simulink model "PC_MSFS_STATION"  (R2021b)
settings: Solver=FixedStepAuto  StartTime=0.0  StopTime=2000  FixedStep=0.03  RelTol=1e-3
undefined symbols (not defined in the file): DiscIntNeverNeededParam, f, MODEL, MODEL_INI
libraries: SimConnectToolbox x11, instrumentlib x7, simulink x5
(part 1 of 2)
settings Model: Creator=Andreas  LastModifiedBy=ccortes9
settings SolverCC: AlgebraicLoopSolver=TrustRegion
settings DebuggingCC: InheritedTsInSrcMsg=none  SFMachineParentedDataDiag=warning

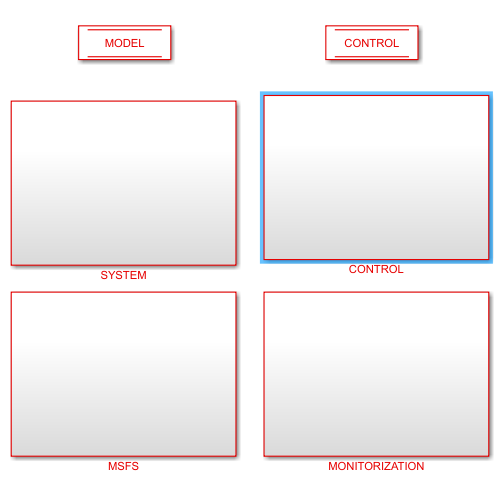
[thumbnail: Simulink's stored preview of the top-level diagram]
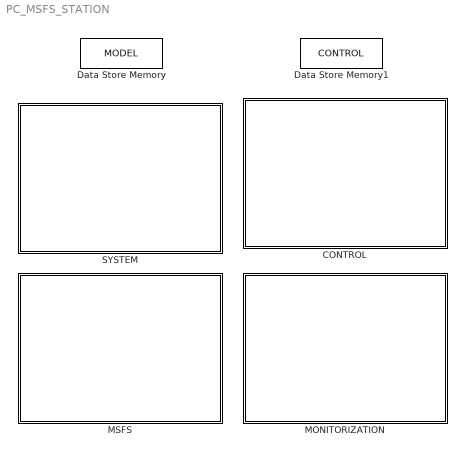
== system PC_MSFS_STATION ==
  CONTROL : Subsystem
  Data Store Memory : DataStoreMemory  DataStoreName=MODEL  ReadBeforeWriteMsg=warning  WriteAfterWriteMsg=warning  WriteAfterReadMsg=warning  InitialValue=MODEL_INI  ShowAdditionalParam=off  OutDataTypeStr=Bus: MODEL_Bus
  Data Store Memory1 : DataStoreMemory  DataStoreName=CONTROL  ReadBeforeWriteMsg=warning  WriteAfterWriteMsg=warning  WriteAfterReadMsg=warning  InitialValue=CONTROL_INI  ShowAdditionalParam=off  OutDataTypeStr=Bus: CONTROL_Bus
  MONITORIZATION : Subsystem
  MSFS : Subsystem
  SYSTEM : Subsystem

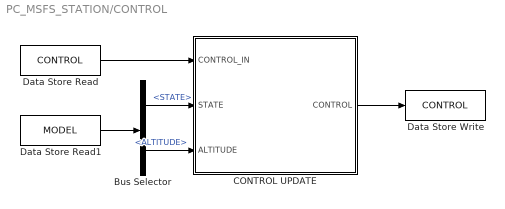
== system PC_MSFS_STATION/CONTROL ==
  Bus Selector : BusSelector  OutputSignals=STATE,INPUT.ALTITUDE
  CONTROL UPDATE : MATLAB Function  TreatAsAtomicUnit=on
  Data Store Read : DataStoreRead  DataStoreName=CONTROL  SampleTime=MODEL_INI.PARAM.SIM_SAMPLING_TIME  IndexOptions=Index vector (dialog)  Indices=1  OutputSizes=1
  Data Store Read1 : DataStoreRead  DataStoreName=MODEL  SampleTime=MODEL_INI.PARAM.SIM_SAMPLING_TIME  IndexOptions=Index vector (dialog)  Indices=1  OutputSizes=1
  Data Store Write : DataStoreWrite  DataStoreName=CONTROL  IndexOptions=Index vector (dialog)  Indices=1  OutputSizes=1
  wires:
  Data Store Read/1 -> CONTROL UPDATE/1(CONTROL_IN)
  CONTROL UPDATE/1(CONTROL) -> Data Store Write/1
  Bus Selector/1 -> CONTROL UPDATE/2(STATE)  "<STATE>"
  Data Store Read1/1 -> Bus Selector/1
  Bus Selector/2 -> CONTROL UPDATE/3(ALTITUDE)  "<ALTITUDE>"

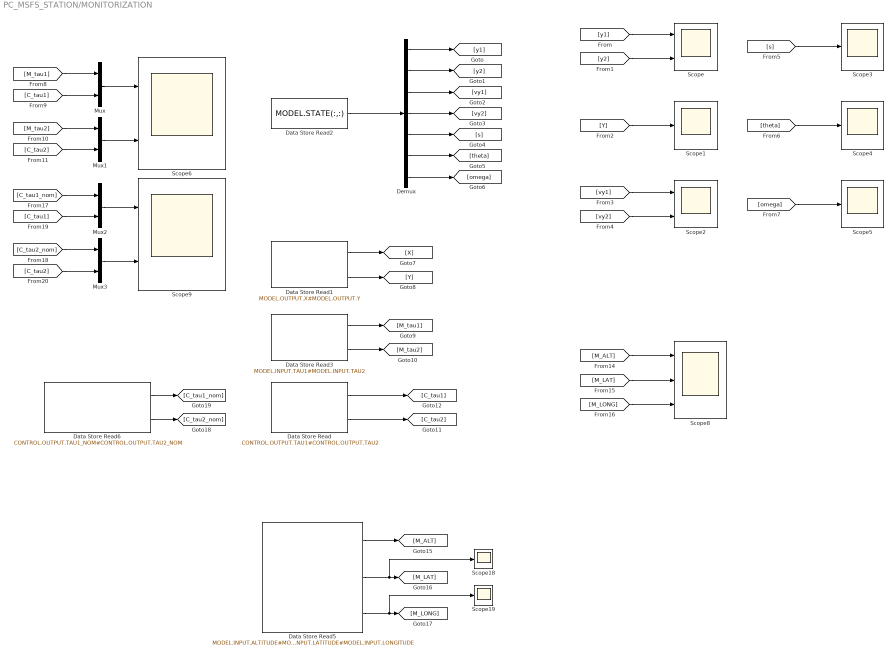
== system PC_MSFS_STATION/MONITORIZATION ==
  Data Store Read : DataStoreRead  DataStoreName=CONTROL  DataStoreElements=CONTROL.OUTPUT.TAU1#CONTROL.OUTPUT.TAU2  IndexOptions=Index vector (dialog)  Indices=1  OutputSizes=1
  Data Store Read1 : DataStoreRead  DataStoreName=MODEL  SampleTime=MODEL_INI.PARAM.SIM_SAMPLING_TIME  DataStoreElements=MODEL.OUTPUT.X#MODEL.OUTPUT.Y  IndexOptions=Index vector (dialog)  Indices=1  OutputSizes=1
  Data Store Read2 : DataStoreRead  DataStoreName=MODEL  SampleTime=MODEL_INI.PARAM.SIM_SAMPLING_TIME  DataStoreElements=MODEL.STATE(:,:)  IndexOptions=Index vector (dialog)  Indices=1  OutputSizes=1
  Data Store Read3 : DataStoreRead  DataStoreName=MODEL  SampleTime=MODEL_INI.PARAM.SIM_SAMPLING_TIME  DataStoreElements=MODEL.INPUT.TAU1#MODEL.INPUT.TAU2  IndexOptions=Index vector (dialog)  Indices=1  OutputSizes=1
  Data Store Read5 : DataStoreRead  DataStoreName=MODEL  SampleTime=MODEL_INI.PARAM.SIM_SAMPLING_TIME  DataStoreElements=MODEL.INPUT.ALTITUDE#MODEL.INPUT.LATITUDE#MODEL.INPUT.LONGITUDE  IndexOptions=Index vector (dialog)  Indices=1  OutputSizes=1
  Data Store Read6 : DataStoreRead  DataStoreName=CONTROL  DataStoreElements=CONTROL.OUTPUT.TAU1_NOM#CONTROL.OUTPUT.TAU2_NOM  IndexOptions=Index vector (dialog)  Indices=1  OutputSizes=1
  Demux : Demux  Outputs=7
  Mux{,1..3} (4 alike) : Mux  Inputs=2
  Scope{,2,6,9} (4 alike) : Scope  NumInputPorts=2
  Scope{1,3..5,18..19} (6 alike) : Scope
  Scope8 : Scope  NumInputPorts=3
  wires:
  Data Store Read2/1 -> Demux/1
  Demux/1 -> [y1]
  Demux/2 -> [y2]
  Demux/3 -> [vy1]
  Demux/4 -> [vy2]
  Demux/5 -> [s]
  Demux/6 -> [theta]
  Demux/7 -> [omega]
  [y1] -> Scope/1
  [y2] -> Scope/2
  Data Store Read1/1 -> [X]
  Data Store Read1/2 -> [Y]
  [Y] -> Scope1/1
  [vy2] -> Scope2/2
  [vy1] -> Scope2/1
  [s] -> Scope3/1
  [theta] -> Scope4/1
  [omega] -> Scope5/1
  Data Store Read3/1 -> [M_tau1]
  Data Store Read3/2 -> [M_tau2]
  Data Store Read/1 -> [C_tau1]
  Data Store Read/2 -> [C_tau2]
  Mux/1 -> Scope6/1
  Mux1/1 -> Scope6/2
  [M_tau1] -> Mux/1
  [M_tau2] -> Mux1/1
  [C_tau2] -> Mux1/2
  [C_tau1] -> Mux/2
  Data Store Read5/2 -> Scope18/1, [M_LAT]
  Data Store Read5/1 -> [M_ALT]
  Data Store Read5/3 -> Scope19/1, [M_LONG]
  [M_LAT] -> Scope8/2
  [M_ALT] -> Scope8/1
  [M_LONG] -> Scope8/3
  Data Store Read6/2 -> [C_tau2_nom]
  Data Store Read6/1 -> [C_tau1_nom]
  [C_tau1] -> Mux2/2
  [C_tau2] -> Mux3/2
  [C_tau2_nom] -> Mux3/1
  [C_tau1_nom] -> Mux2/1
  Mux3/1 -> Scope9/2
  Mux2/1 -> Scope9/1

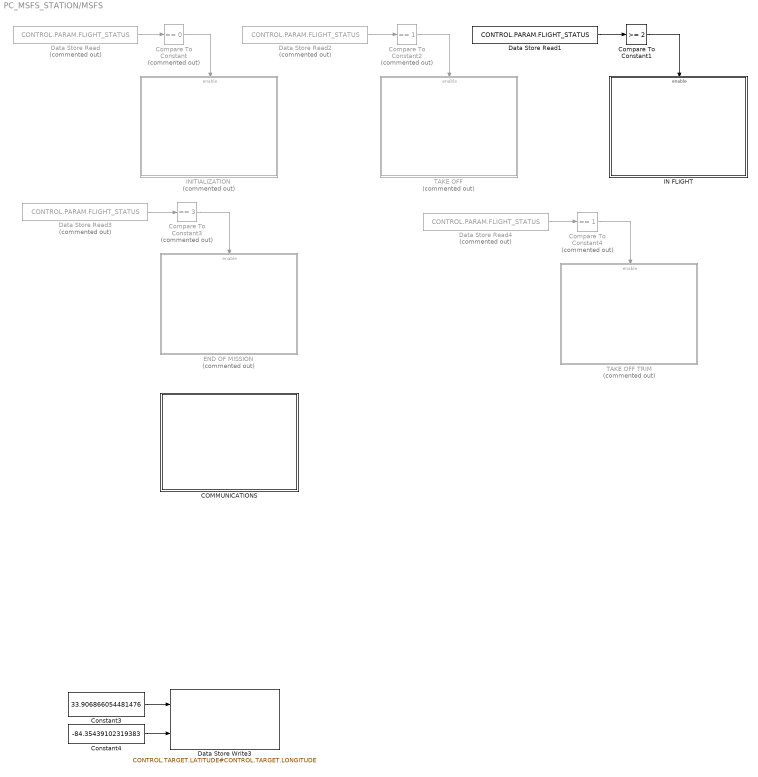
== system PC_MSFS_STATION/MSFS ==
  COMMUNICATIONS : Subsystem
  Compare To Constant : simulink/Logic and Bit Operations/Compare To Constant  Commented=on  relop===  const=0  OutDataTypeStr=boolean
  Compare To Constant1 : simulink/Logic and Bit Operations/Compare To Constant  relop=>=  const=2  OutDataTypeStr=boolean
  Compare To Constant2 : simulink/Logic and Bit Operations/Compare To Constant  Commented=on  relop===  const=1  OutDataTypeStr=boolean
  Compare To Constant3 : simulink/Logic and Bit Operations/Compare To Constant  Commented=on  relop===  const=3  OutDataTypeStr=boolean
  Compare To Constant4 : simulink/Logic and Bit Operations/Compare To Constant  Commented=on  relop===  const=1  OutDataTypeStr=boolean
  Constant3 : Constant  Value=33.906866054481476  SampleTime=-1
  Constant4 : Constant  Value=-84.35439102319383  SampleTime=-1
  Data Store Read{,2..4} (4 alike) : DataStoreRead  Commented=on  DataStoreName=CONTROL  DataStoreElements=CONTROL.PARAM.FLIGHT_STATUS  IndexOptions=Index vector (dialog)  Indices=1  OutputSizes=1
  Data Store Read1 : DataStoreRead  DataStoreName=CONTROL  DataStoreElements=CONTROL.PARAM.FLIGHT_STATUS  IndexOptions=Index vector (dialog)  Indices=1  OutputSizes=1
  Data Store Write3 : DataStoreWrite  DataStoreName=CONTROL  DataStoreElements=CONTROL.TARGET.LATITUDE#CONTROL.TARGET.LONGITUDE  IndexOptions=Index vector (dialog)  Indices=1  OutputSizes=1
  END OF MISSION : Subsystem  Commented=on
  IN FLIGHT : Subsystem
  INITIALIZATION : Subsystem  Commented=on
  TAKE OFF : Subsystem  Commented=on
  TAKE OFF TRIM : Subsystem  Commented=on
  wires:
  Data Store Read/1 -> Compare To Constant/1
  Compare To Constant/1 -> INITIALIZATION/Enable
  Data Store Read1/1 -> Compare To Constant1/1
  Data Store Read2/1 -> Compare To Constant2/1
  Compare To Constant2/1 -> TAKE OFF/Enable
  Compare To Constant3/1 -> END OF MISSION/Enable
  Data Store Read3/1 -> Compare To Constant3/1
  Data Store Read4/1 -> Compare To Constant4/1
  Compare To Constant4/1 -> TAKE OFF TRIM/Enable
  Constant3/1 -> Data Store Write3/1
  Constant4/1 -> Data Store Write3/2
  Compare To Constant1/1 -> IN FLIGHT/Enable

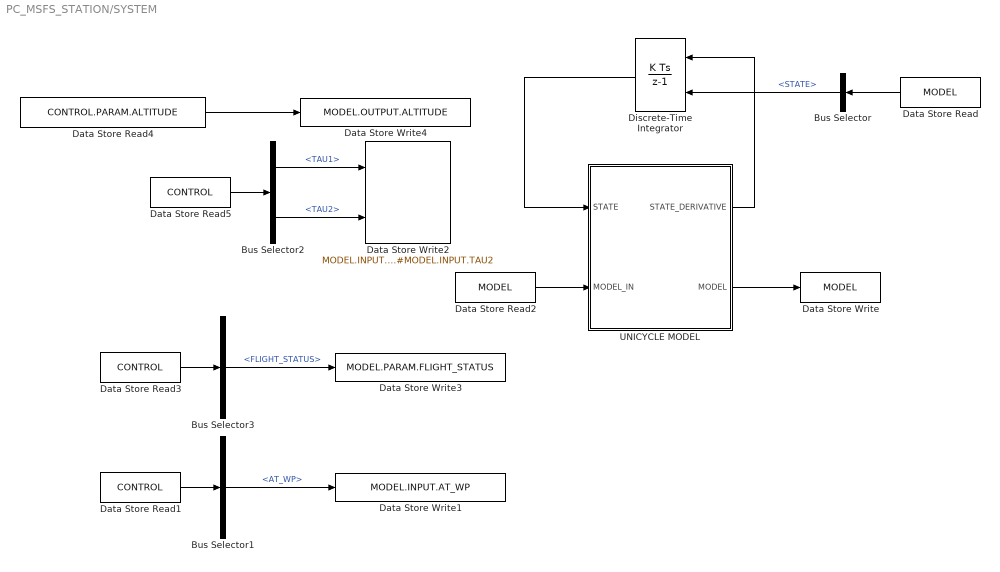
== system PC_MSFS_STATION/SYSTEM ==
  Bus Selector : BusSelector  OutputSignals=STATE
  Bus Selector1 : BusSelector  OutputSignals=OUTPUT.AT_WP
  Bus Selector2 : BusSelector  OutputSignals=OUTPUT.TAU1,OUTPUT.TAU2
  Bus Selector3 : BusSelector  OutputSignals=PARAM.FLIGHT_STATUS
  Data Store Read : DataStoreRead  DataStoreName=MODEL  SampleTime=MODEL_INI.PARAM.SIM_SAMPLING_TIME  IndexOptions=Index vector (dialog)  Indices=1  OutputSizes=1
  Data Store Read1 : DataStoreRead  DataStoreName=CONTROL  IndexOptions=Index vector (dialog)  Indices=1  OutputSizes=1
  Data Store Read2 : DataStoreRead  DataStoreName=MODEL  SampleTime=MODEL_INI.PARAM.SIM_SAMPLING_TIME  IndexOptions=Index vector (dialog)  Indices=1  OutputSizes=1
  Data Store Read3 : DataStoreRead  DataStoreName=CONTROL  IndexOptions=Index vector (dialog)  Indices=1  OutputSizes=1
  Data Store Read4 : DataStoreRead  DataStoreName=CONTROL  DataStoreElements=CONTROL.PARAM.ALTITUDE  IndexOptions=Index vector (dialog)  Indices=1  OutputSizes=1
  Data Store Read5 : DataStoreRead  DataStoreName=CONTROL  IndexOptions=Index vector (dialog)  Indices=1  OutputSizes=1
  Data Store Write : DataStoreWrite  DataStoreName=MODEL  IndexOptions=Index vector (dialog)  Indices=1  OutputSizes=1
  Data Store Write1 : DataStoreWrite  DataStoreName=MODEL  DataStoreElements=MODEL.INPUT.AT_WP  IndexOptions=Index vector (dialog)  Indices=1  OutputSizes=1
  Data Store Write2 : DataStoreWrite  DataStoreName=MODEL  DataStoreElements=MODEL.INPUT.TAU1#MODEL.INPUT.TAU2  IndexOptions=Index vector (dialog)  Indices=1  OutputSizes=1
  Data Store Write3 : DataStoreWrite  DataStoreName=MODEL  DataStoreElements=MODEL.PARAM.FLIGHT_STATUS  IndexOptions=Index vector (dialog)  Indices=1  OutputSizes=1
  Data Store Write4 : DataStoreWrite  DataStoreName=MODEL  DataStoreElements=MODEL.OUTPUT.ALTITUDE  IndexOptions=Index vector (dialog)  Indices=1  OutputSizes=1
  Discrete-Time Integrator : DiscreteIntegrator  InitialConditionSource=external  SampleTime=-1  ICPrevOutput=DiscIntNeverNeededParam  ICPrevScaledInput=DiscIntNeverNeededParam
  UNICYCLE MODEL : MATLAB Function  TreatAsAtomicUnit=on
  wires:
  Discrete-Time Integrator/1 -> UNICYCLE MODEL/1(STATE)
  UNICYCLE MODEL/1(STATE_DERIVATIVE) -> Discrete-Time Integrator/1
  Bus Selector/1 -> Discrete-Time Integrator/2  "<STATE>"
  Data Store Read/1 -> Bus Selector/1
  Data Store Read2/1 -> UNICYCLE MODEL/2(MODEL_IN)
  UNICYCLE MODEL/2(MODEL) -> Data Store Write/1
  Bus Selector2/2 -> Data Store Write2/2  "<TAU2>"
  Bus Selector2/1 -> Data Store Write2/1  "<TAU1>"
  Data Store Read5/1 -> Bus Selector2/1
  Data Store Read3/1 -> Bus Selector3/1
  Bus Selector3/1 -> Data Store Write3/1  "<FLIGHT_STATUS>"
  Data Store Read4/1 -> Data Store Write4/1
  Bus Selector1/1 -> Data Store Write1/1  "<AT_WP>"
  Data Store Read1/1 -> Bus Selector1/1

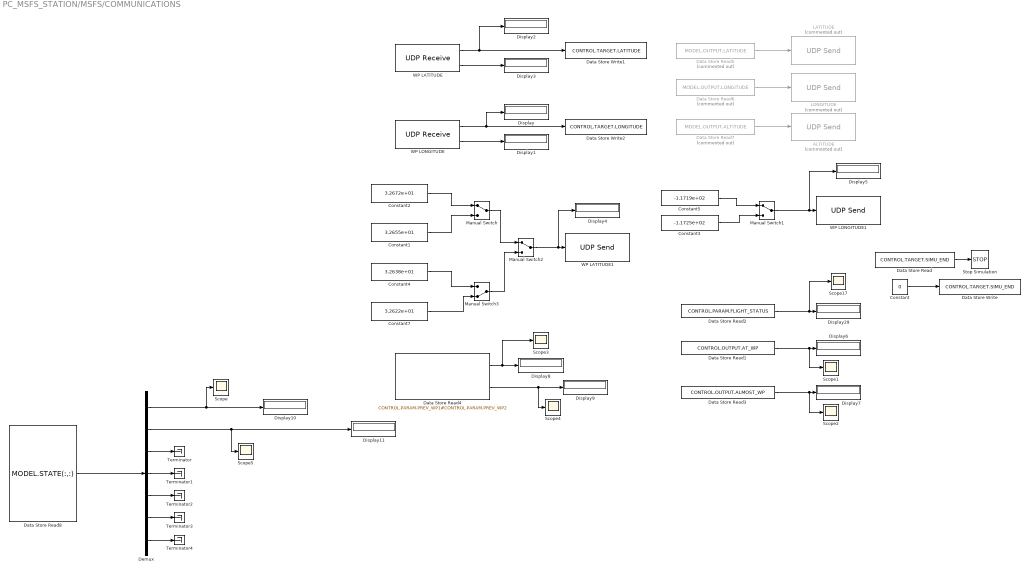
== system PC_MSFS_STATION/MSFS/COMMUNICATIONS ==
  ALTITUDE : instrumentlib/UDP Send  Commented=on  Host=127.0.0.1  Port=8082  LocalPort=8085  EnablePortSharing=off  ByteOrder=BigEndian  OutputDatagramPacketSize=512  EnableBlockingMode=on  LocalAddress=127.0.0.1
  Constant : Constant  Value=0  SampleTime=-1
  Constant1 : Constant  Value=3.2655e+01  SampleTime=0.03
  Constant2 : Constant  Value=3.2672e+01  SampleTime=0.03
  Constant3 : Constant  Value=-1.1725e+02  SampleTime=0.03
  Constant4 : Constant  Value=3.2638e+01  SampleTime=0.03
  Constant5 : Constant  Value=-1.1719e+02  SampleTime=0.03
  Constant7 : Constant  Value=3.2622e+01  SampleTime=0.03
  Data Store Read : DataStoreRead  DataStoreName=CONTROL  DataStoreElements=CONTROL.TARGET.SIMU_END  IndexOptions=Index vector (dialog)  Indices=1  OutputSizes=1
  Data Store Read1 : DataStoreRead  DataStoreName=CONTROL  DataStoreElements=CONTROL.OUTPUT.AT_WP  IndexOptions=Index vector (dialog)  Indices=1  OutputSizes=1
  Data Store Read2 : DataStoreRead  DataStoreName=CONTROL  DataStoreElements=CONTROL.PARAM.FLIGHT_STATUS  IndexOptions=Index vector (dialog)  Indices=1  OutputSizes=1
  Data Store Read3 : DataStoreRead  DataStoreName=CONTROL  DataStoreElements=CONTROL.OUTPUT.ALMOST_WP  IndexOptions=Index vector (dialog)  Indices=1  OutputSizes=1
  Data Store Read4 : DataStoreRead  DataStoreName=CONTROL  DataStoreElements=CONTROL.PARAM.PREV_WP1#CONTROL.PARAM.PREV_WP2  IndexOptions=Index vector (dialog)  Indices=1  OutputSizes=1
  Data Store Read5 : DataStoreRead  Commented=on  DataStoreName=MODEL  DataStoreElements=MODEL.OUTPUT.LATITUDE  IndexOptions=Index vector (dialog)  Indices=1  OutputSizes=1
  Data Store Read6 : DataStoreRead  Commented=on  DataStoreName=MODEL  DataStoreElements=MODEL.OUTPUT.LONGITUDE  IndexOptions=Index vector (dialog)  Indices=1  OutputSizes=1
  Data Store Read7 : DataStoreRead  Commented=on  DataStoreName=MODEL  DataStoreElements=MODEL.OUTPUT.ALTITUDE  IndexOptions=Index vector (dialog)  Indices=1  OutputSizes=1
  Data Store Read8 : DataStoreRead  DataStoreName=MODEL  SampleTime=MODEL_INI.PARAM.SIM_SAMPLING_TIME  DataStoreElements=MODEL.STATE(:,:)  IndexOptions=Index vector (dialog)  Indices=1  OutputSizes=1
  Data Store Write : DataStoreWrite  DataStoreName=CONTROL  DataStoreElements=CONTROL.TARGET.SIMU_END  IndexOptions=Index vector (dialog)  Indices=1  OutputSizes=1
  Data Store Write1 : DataStoreWrite  DataStoreName=CONTROL  DataStoreElements=CONTROL.TARGET.LATITUDE  IndexOptions=Index vector (dialog)  Indices=1  OutputSizes=1
  Data Store Write2 : DataStoreWrite  DataStoreName=CONTROL  DataStoreElements=CONTROL.TARGET.LONGITUDE  IndexOptions=Index vector (dialog)  Indices=1  OutputSizes=1
  Demux : Demux  Outputs=7
  Display{,1..11,29} (13 alike) : Display
  LATITUDE : instrumentlib/UDP Send  Commented=on  Host=127.0.0.1  Port=8086  LocalPort=8081  EnablePortSharing=off  ByteOrder=BigEndian  OutputDatagramPacketSize=512  EnableBlockingMode=on  LocalAddress=127.0.0.1
  LONGITUDE : instrumentlib/UDP Send  Commented=on  Host=127.0.0.1  Port=8084  LocalPort=8083  EnablePortSharing=off  ByteOrder=BigEndian  OutputDatagramPacketSize=512  EnableBlockingMode=on  LocalAddress=127.0.0.1
  Manual Switch : ManualSwitch
  Manual Switch1 : ManualSwitch
  Manual Switch2 : ManualSwitch
  Manual Switch3 : ManualSwitch  CurrentSetting=0
  Scope{,1..5,17} (7 alike) : Scope
  Stop Simulation : Stop
  Terminator{,1..4} (5 alike) : Terminator
  WP LATITUDE : instrumentlib/UDP Receive  Host=127.0.0.1  Port=8087  LocalPort=8080  EnablePortSharing=off  GetLatestData=off  DataSize=[1 1]  DataType=double  ASCIIFormatting=%f,  Terminator=LF  ByteOrder=BigEndian  EnableBlockingMode=off  Timeout=10  SampleTime=-1  LocalAddress=127.0.0.1
  WP LATITUDE1 : instrumentlib/UDP Send  Host=127.0.0.1  Port=8080  LocalPort=8087  EnablePortSharing=off  ByteOrder=BigEndian  OutputDatagramPacketSize=512  EnableBlockingMode=on  LocalAddress=127.0.0.1
  WP LONGITUDE : instrumentlib/UDP Receive  Host=127.0.0.1  Port=8089  LocalPort=8088  EnablePortSharing=off  GetLatestData=off  DataSize=[1 1]  DataType=double  ASCIIFormatting=%f,  Terminator=LF  ByteOrder=BigEndian  EnableBlockingMode=off  Timeout=10  SampleTime=-1  LocalAddress=127.0.0.1
  WP LONGITUDE1 : instrumentlib/UDP Send  Host=127.0.0.1  Port=8088  LocalPort=8089  EnablePortSharing=off  ByteOrder=BigEndian  OutputDatagramPacketSize=512  EnableBlockingMode=on  LocalAddress=127.0.0.1
  wires:
  WP LONGITUDE/1 -> Data Store Write2/1, Display/1
  WP LATITUDE/2 -> Display3/1
  WP LATITUDE/1 -> Display2/1, Data Store Write1/1
  Data Store Read6/1 -> LONGITUDE/1
  Data Store Read7/1 -> ALTITUDE/1
  Data Store Read5/1 -> LATITUDE/1
  WP LONGITUDE/2 -> Display1/1
  Constant5/1 -> Manual Switch1/1
  Constant2/1 -> Manual Switch/1
  Constant1/1 -> Manual Switch/2
  Constant3/1 -> Manual Switch1/2
  Manual Switch1/1 -> Display5/1, WP LONGITUDE1/1
  Manual Switch/1 -> Manual Switch2/1
  Manual Switch2/1 -> Display4/1, WP LATITUDE1/1
  Constant4/1 -> Manual Switch3/1
  Constant7/1 -> Manual Switch3/2
  Manual Switch3/1 -> Manual Switch2/2
  Data Store Read1/1 -> Scope1/1, Display6/1
  Data Store Read2/1 -> Scope17/1, Display29/1
  Data Store Read3/1 -> Scope2/1, Display7/1
  Data Store Read4/1 -> Scope3/1, Display8/1
  Data Store Read4/2 -> Scope4/1, Display9/1
  Constant/1 -> Data Store Write/1
  Data Store Read/1 -> Stop Simulation/1
  Data Store Read8/1 -> Demux/1
  Demux/1 -> Scope/1, Display10/1
  Demux/2 -> Scope5/1, Display11/1
  Demux/3 -> Terminator/1
  Demux/4 -> Terminator1/1
  Demux/5 -> Terminator2/1
  Demux/6 -> Terminator3/1
  Demux/7 -> Terminator4/1

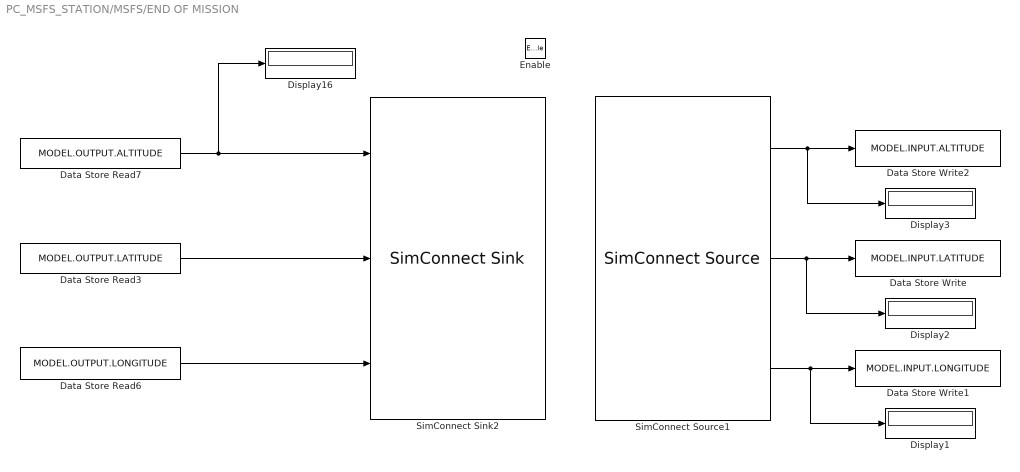
== system PC_MSFS_STATION/MSFS/END OF MISSION ==
  Enable : EnablePort
  Data Store Read3 : DataStoreRead  DataStoreName=MODEL  DataStoreElements=MODEL.OUTPUT.LATITUDE  IndexOptions=Index vector (dialog)  Indices=1  OutputSizes=1
  Data Store Read6 : DataStoreRead  DataStoreName=MODEL  DataStoreElements=MODEL.OUTPUT.LONGITUDE  IndexOptions=Index vector (dialog)  Indices=1  OutputSizes=1
  Data Store Read7 : DataStoreRead  DataStoreName=MODEL  DataStoreElements=MODEL.OUTPUT.ALTITUDE  IndexOptions=Index vector (dialog)  Indices=1  OutputSizes=1
  Data Store Write : DataStoreWrite  DataStoreName=MODEL  DataStoreElements=MODEL.INPUT.LATITUDE  IndexOptions=Index vector (dialog)  Indices=1  OutputSizes=1
  Data Store Write1 : DataStoreWrite  DataStoreName=MODEL  DataStoreElements=MODEL.INPUT.LONGITUDE  IndexOptions=Index vector (dialog)  Indices=1  OutputSizes=1
  Data Store Write2 : DataStoreWrite  DataStoreName=MODEL  DataStoreElements=MODEL.INPUT.ALTITUDE  IndexOptions=Index vector (dialog)  Indices=1  OutputSizes=1
  Display{1..3,16} (4 alike) : Display
  SimConnect Sink2 : SimConnectToolbox/SimConnect Sink  configurationIndex=0  connectionName=SimConnectSink  variables=|
      | PLANE ALTITUDE, FEET;
      | PLANE LATITUDE, RADIANS;
      | PLANE LONGITUDE, RADIANS;
      settings: SourceProductName=SimConnect Toolbox
      mask Display:
      | % This is a new mask on top of the base mask.
      | % Use "View base mask" link below to see the base mask.
      | %port_label('input', 1, 'Rudder Trim', 'texmode', 'on')
      | port_label('input', 1, 'PLANE ALTITUDE, FEET', 'texmode', 'on')
      | port_label('input', 2, 'PLANE LATITUDE, RADIANS', 'texmode', 'on')
      | port_label('input', 3, 'PLANE LONGITUDE, RADIANS', 'texmode', 'on')
  SimConnect Source1 : SimConnectToolbox/SimConnect Source  configurationIndex=0  connectionName=SimConnectSource  variables=|
      | PLANE ALTITUDE, FEET;
      | PLANE LATITUDE, RADIANS;
      | PLANE LONGITUDE, RADIANS;
      settings: SourceProductName=SimConnect Toolbox
      mask Display:
      | % This is a new mask on top of the base mask.
      | % Use "View base mask" link below to see the base mask.
      | % port_label('output', 1, 'g', 'texmode', 'on')
      | port_label('output', 1, 'PLANE ALTITUDE, FEET', 'texmode', 'on')
      | port_label('output', 2, 'PLANE LATITUDE, RADIANS', 'texmode', 'on')
      | port_label('output', 3, 'PLANE LONGITUDE, RADIANS', 'texmode', 'on')
  wires:
  SimConnect Source1/3 -> Data Store Write1/1, Display1/1
  SimConnect Source1/1 -> Data Store Write2/1, Display3/1
  SimConnect Source1/2 -> Display2/1, Data Store Write/1
  Data Store Read7/1 -> Display16/1, SimConnect Sink2/1
  Data Store Read6/1 -> SimConnect Sink2/3
  Data Store Read3/1 -> SimConnect Sink2/2

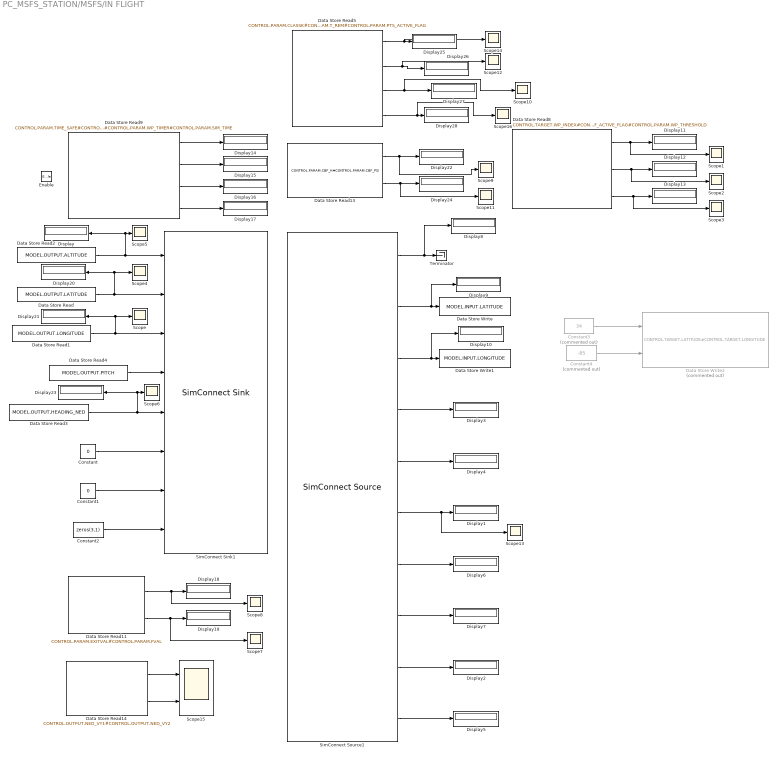
== system PC_MSFS_STATION/MSFS/IN FLIGHT ==
  Enable : EnablePort
  Constant : Constant  Value=0  SampleTime=-1
  Constant1 : Constant  Value=0  SampleTime=-1
  Constant2 : Constant  Value=zeros(3,1)  SampleTime=-1
  Constant3 : Constant  Commented=on  Value=34
  Constant4 : Constant  Commented=on  Value=-85
  Data Store Read : DataStoreRead  DataStoreName=MODEL  DataStoreElements=MODEL.OUTPUT.LATITUDE  IndexOptions=Index vector (dialog)  Indices=1  OutputSizes=1
  Data Store Read1 : DataStoreRead  DataStoreName=MODEL  DataStoreElements=MODEL.OUTPUT.LONGITUDE  IndexOptions=Index vector (dialog)  Indices=1  OutputSizes=1
  Data Store Read11 : DataStoreRead  DataStoreName=CONTROL  DataStoreElements=CONTROL.PARAM.EXITVAL#CONTROL.PARAM.FVAL  IndexOptions=Index vector (dialog)  Indices=1  OutputSizes=1
  Data Store Read13 : DataStoreRead  DataStoreName=CONTROL  DataStoreElements=CONTROL.PARAM.CBF_H#CONTROL.PARAM.CBF_PSI  IndexOptions=Index vector (dialog)  Indices=1  OutputSizes=1
  Data Store Read14 : DataStoreRead  DataStoreName=CONTROL  DataStoreElements=CONTROL.OUTPUT.NED_VY1#CONTROL.OUTPUT.NED_VY2  IndexOptions=Index vector (dialog)  Indices=1  OutputSizes=1
  Data Store Read2 : DataStoreRead  DataStoreName=MODEL  DataStoreElements=MODEL.OUTPUT.ALTITUDE  IndexOptions=Index vector (dialog)  Indices=1  OutputSizes=1
  Data Store Read3 : DataStoreRead  DataStoreName=MODEL  DataStoreElements=MODEL.OUTPUT.HEADING_NED  IndexOptions=Index vector (dialog)  Indices=1  OutputSizes=1
  Data Store Read4 : DataStoreRead  DataStoreName=MODEL  DataStoreElements=MODEL.OUTPUT.PITCH  IndexOptions=Index vector (dialog)  Indices=1  OutputSizes=1
  Data Store Read5 : DataStoreRead  DataStoreName=CONTROL  DataStoreElements=CONTROL.PARAM.CLASSK#CONTROL.PARAM.MU2#CONTROL.PARAM.T_REM#CONTROL.PARAM.PTS_ACTIVE_FLAG  IndexOptions=Index vector (dialog)  Indices=1  OutputSizes=1
  Data Store Read8 : DataStoreRead  DataStoreName=CONTROL  DataStoreElements=CONTROL.TARGET.WP_INDEX#CONTROL.PARAM.CBF_ACTIVE_FLAG#CONTROL.PARAM.WP_THRESHOLD  IndexOptions=Index vector (dialog)  Indices=1  OutputSizes=1
  Data Store Read9 : DataStoreRead  DataStoreName=CONTROL  DataStoreElements=CONTROL.PARAM.TIME_SAFE#CONTROL.PARAM.TIMER#CONTROL.PARAM.WP_TIMER#CONTROL.PARAM.SIM_TIME  IndexOptions=Index vector (dialog)  Indices=1  OutputSizes=1
  Data Store Write : DataStoreWrite  DataStoreName=MODEL  DataStoreElements=MODEL.INPUT.LATITUDE  IndexOptions=Index vector (dialog)  Indices=1  OutputSizes=1
  Data Store Write1 : DataStoreWrite  DataStoreName=MODEL  DataStoreElements=MODEL.INPUT.LONGITUDE  IndexOptions=Index vector (dialog)  Indices=1  OutputSizes=1
  Data Store Write2 : DataStoreWrite  Commented=on  DataStoreName=CONTROL  DataStoreElements=CONTROL.TARGET.LATITUDE#CONTROL.TARGET.LONGITUDE  IndexOptions=Index vector (dialog)  Indices=1  OutputSizes=1
  Display{,1..28} (29 alike) : Display
  Scope{,1..14,16} (16 alike) : Scope
  Scope15 : Scope  NumInputPorts=2
  SimConnect Sink1 : SimConnectToolbox/SimConnect Sink  configurationIndex=0  connectionName=SimConnectSink  variables=|
      | PLANE ALTITUDE, FEET;
      | PLANE LATITUDE, RADIANS;
      | PLANE LONGITUDE, RADIANS;
      | PLANE PITCH DEGREES, RADIANS;
      | PLANE HEADING DEGREES TRUE, RADIANS;
      | ROTATION VELOCITY BODY X, FEET PER SECOND;
      | AILERON POSITION, POSITION;
      | AILERON TRIM PCT, PERCENT;
      settings: SourceProductName=SimConnect Toolbox
      mask Display:
      | % This is a new mask on top of the base mask.
      | % Use "View base mask" link below to see the base mask.
      | %port_label('input', 1, 'Rudder Trim', 'texmode', 'on')
      | port_label('input', 1, 'PLANE ALTITUDE, FEET', 'texmode', 'on')
      | port_label('input', 2, 'PLANE LATITUDE, RADIANS', 'texmode', 'on')
      | port_label('input', 3, 'PLANE LONGITUDE, RADIANS', 'texmode', 'on')
      | port_label('input', 4, 'PITCH DEGREES, RADIANS', 'texmode', 'on')
      | port_label('input', 5, 'HEADING DEGREES TRUE, RADIANS', 'texmode', 'on')
      | port_label('input', 6, 'VELOCITY BODY X, FEET PER SECOND', 'texmode', 'on')
      | port_label('input', 7, 'AILERON POSITION, POSITION', 'texmode', 'on')
      | port_label('input', 8, 'AILERON TRIM PCT, PERCENT OVER 100', 'texmode', 'on')
  SimConnect Source1 : SimConnectToolbox/SimConnect Source  configurationIndex=0  connectionName=SimConnectSource  variables=|
      | PLANE ALTITUDE, FEET;
      | PLANE LATITUDE, RADIANS;
      | PLANE LONGITUDE, RADIANS;
      | ROTATION VELOCITY BODY X, FEET PER SECOND;
      | PLANE PITCH DEGREES, RADIANS;
      | PLANE HEADING DEGREES TRUE, RADIANS;
      | PLANE HEADING DEGREES MAGNETIC, RADIANS;
      | PLANE HEADING DEGREES GYRO, DEGREES;
      | AILERON POSITION, POSITION;
      | AILERON TRIM PCT, PERCENT OVER 100;
      settings: SourceProductName=SimConnect Toolbox
      mask Display:
      | % This is a new mask on top of the base mask.
      | % Use "View base mask" link below to see the base mask.
      | % port_label('output', 1, 'g', 'texmode', 'on')
      | port_label('output', 1, 'PLANE ALTITUDE, FEET', 'texmode', 'on')
      | port_label('output', 2, 'PLANE LATITUDE, RADIANS', 'texmode', 'on')
      | port_label('output', 3, 'PLANE LONGITUDE, RADIANS', 'texmode', 'on')
      | port_label('output', 4, 'VELOCITY BODY X, FEET PER SECOND', 'texmode', 'on')
      | port_label('output', 5, 'PITCH DEGREES, RADIANS', 'texmode', 'on')
      | port_label('output', 6, 'HEADING DEGREES TRUE, RADIANS', 'texmode', 'on')
      | port_label('output', 7, 'HEADING DEGREES MAGNETIC, RADIANS', 'texmode', 'on')
      | port_label('output', 8, 'HEADING DEGREES GYRO, DEGREES', 'texmode', 'on')
      | port_label('output', 9, 'AILERON POSITION, POSITION', 'texmode', 'on')
      | port_label('output', 10, 'AILERON TRIM PCT, PERCENT OVER 100', 'texmode', 'on')
  Terminator : Terminator
  wires:
  Constant2/1 -> SimConnect Sink1/8
  SimConnect Source1/9 -> Display2/1
  Constant/1 -> SimConnect Sink1/6
  Data Store Read1/1 -> Display21/1, Scope/1, SimConnect Sink1/3
  Constant1/1 -> SimConnect Sink1/7
  SimConnect Source1/5 -> Display4/1
  SimConnect Source1/3 -> Display10/1, Data Store Write1/1
  SimConnect Source1/2 -> Display9/1, Data Store Write/1
  SimConnect Source1/8 -> Display7/1
  SimConnect Source1/6 -> Scope13/1, Display1/1
  Data Store Read2/1 -> Display/1, Scope5/1, SimConnect Sink1/1
  Data Store Read/1 -> Display20/1, Scope4/1, SimConnect Sink1/2
  Data Store Read4/1 -> SimConnect Sink1/4
  SimConnect Source1/4 -> Display3/1
  SimConnect Source1/1 -> Terminator/1, Display8/1
  SimConnect Source1/7 -> Display6/1
  SimConnect Source1/10 -> Display5/1
  Data Store Read9/1 -> Display14/1
  Data Store Read9/2 -> Display15/1
  Data Store Read9/3 -> Display16/1
  Data Store Read9/4 -> Display17/1
  Data Store Read13/1 -> Scope9/1, Display22/1
  Data Store Read13/2 -> Scope11/1, Display24/1
  Data Store Read14/1 -> Scope15/1
  Data Store Read14/2 -> Scope15/2
  Data Store Read11/1 -> Scope8/1, Display18/1
  Data Store Read11/2 -> Scope7/1, Display19/1
  Data Store Read8/1 -> Scope1/1, Display11/1
  Data Store Read8/2 -> Display12/1, Scope2/1
  Data Store Read8/3 -> Display13/1, Scope3/1
  Data Store Read3/1 -> Display23/1, Scope6/1, SimConnect Sink1/5
  Data Store Read5/1 -> Display25/1, Scope14/1
  Data Store Read5/2 -> Display26/1, Scope12/1
  Data Store Read5/3 -> Scope10/1, Display27/1
  Data Store Read5/4 -> Scope16/1, Display28/1
  Constant3/1 -> Data Store Write2/1
  Constant4/1 -> Data Store Write2/2

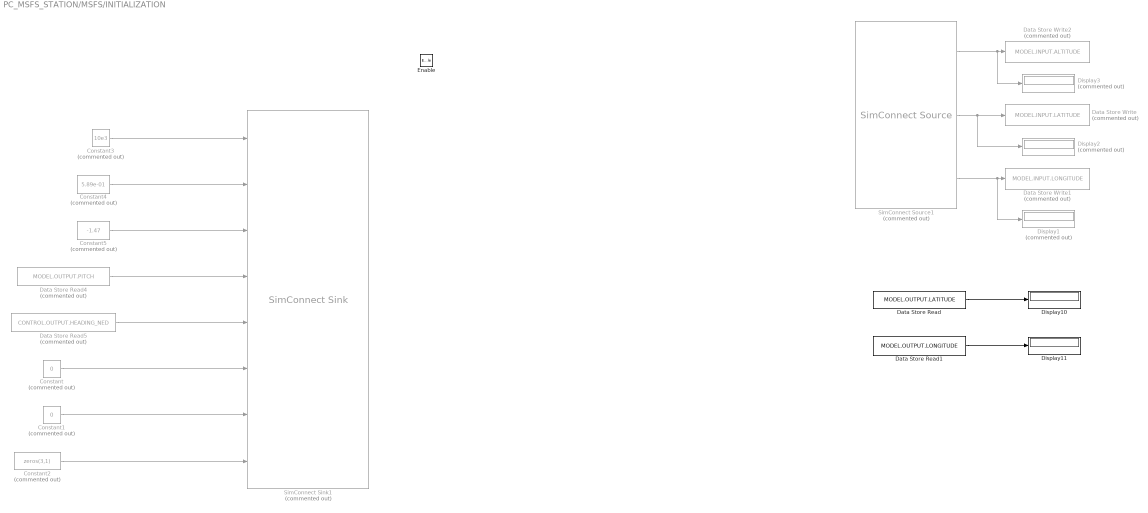
== system PC_MSFS_STATION/MSFS/INITIALIZATION ==
  Enable : EnablePort
  Constant : Constant  Commented=on  Value=0  SampleTime=-1
  Constant1 : Constant  Commented=on  Value=0  SampleTime=-1
  Constant2 : Constant  Commented=on  Value=zeros(3,1)  SampleTime=-1
  Constant3 : Constant  Commented=on  Value=10e3  SampleTime=-1
  Constant4 : Constant  Commented=on  Value=5.89e-01  SampleTime=-1
  Constant5 : Constant  Commented=on  Value=-1.47  SampleTime=-1
  Data Store Read : DataStoreRead  DataStoreName=MODEL  DataStoreElements=MODEL.OUTPUT.LATITUDE  IndexOptions=Index vector (dialog)  Indices=1  OutputSizes=1
  Data Store Read1 : DataStoreRead  DataStoreName=MODEL  DataStoreElements=MODEL.OUTPUT.LONGITUDE  IndexOptions=Index vector (dialog)  Indices=1  OutputSizes=1
  Data Store Read4 : DataStoreRead  Commented=on  DataStoreName=MODEL  DataStoreElements=MODEL.OUTPUT.PITCH  IndexOptions=Index vector (dialog)  Indices=1  OutputSizes=1
  Data Store Read5 : DataStoreRead  Commented=on  DataStoreName=CONTROL  DataStoreElements=CONTROL.OUTPUT.HEADING_NED  IndexOptions=Index vector (dialog)  Indices=1  OutputSizes=1
  Data Store Write : DataStoreWrite  Commented=on  DataStoreName=MODEL  DataStoreElements=MODEL.INPUT.LATITUDE  IndexOptions=Index vector (dialog)  Indices=1  OutputSizes=1
  Data Store Write1 : DataStoreWrite  Commented=on  DataStoreName=MODEL  DataStoreElements=MODEL.INPUT.LONGITUDE  IndexOptions=Index vector (dialog)  Indices=1  OutputSizes=1
  Data Store Write2 : DataStoreWrite  Commented=on  DataStoreName=MODEL  DataStoreElements=MODEL.INPUT.ALTITUDE  IndexOptions=Index vector (dialog)  Indices=1  OutputSizes=1
  Display1 : Display  Commented=on
  Display10 : Display
  Display11 : Display
  Display2 : Display  Commented=on
  Display3 : Display  Commented=on
  SimConnect Sink1 : SimConnectToolbox/SimConnect Sink  Commented=on  configurationIndex=0  connectionName=SimConnectSink  variables=|
      | PLANE ALTITUDE, FEET;
      | PLANE LATITUDE, RADIANS;
      | PLANE LONGITUDE, RADIANS;
      | PLANE PITCH DEGREES, RADIANS;
      | PLANE HEADING DEGREES TRUE, RADIANS;
      | ROTATION VELOCITY BODY X, FEET PER SECOND;
      | AILERON POSITION, POSITION;
      | AILERON TRIM PCT, PERCENT;
      settings: SourceProductName=SimConnect Toolbox
      mask Display:
      | % This is a new mask on top of the base mask.
      | % Use "View base mask" link below to see the base mask.
      | %port_label('input', 1, 'Rudder Trim', 'texmode', 'on')
      | port_label('input', 1, 'PLANE ALTITUDE, FEET', 'texmode', 'on')
      | port_label('input', 2, 'PLANE LATITUDE, RADIANS', 'texmode', 'on')
      | port_label('input', 3, 'PLANE LONGITUDE, RADIANS', 'texmode', 'on')
      | port_label('input', 4, 'PITCH DEGREES, RADIANS', 'texmode', 'on')
      | port_label('input', 5, 'HEADING DEGREES TRUE, RADIANS', 'texmode', 'on')
      | port_label('input', 6, 'VELOCITY BODY X, FEET PER SECOND', 'texmode', 'on')
      | port_label('input', 7, 'AILERON POSITION, POSITION', 'texmode', 'on')
      | port_label('input', 8, 'AILERON TRIM PCT, PERCENT OVER 100', 'texmode', 'on')
  SimConnect Source1 : SimConnectToolbox/SimConnect Source  Commented=on  configurationIndex=0  connectionName=SimConnectSource  variables=|
      | PLANE ALTITUDE, FEET;
      | PLANE LATITUDE, RADIANS;
      | PLANE LONGITUDE, RADIANS;
      settings: SourceProductName=SimConnect Toolbox
      mask Display:
      | % This is a new mask on top of the base mask.
      | % Use "View base mask" link below to see the base mask.
      | % port_label('output', 1, 'g', 'texmode', 'on')
      | port_label('output', 1, 'PLANE ALTITUDE, FEET', 'texmode', 'on')
      | port_label('output', 2, 'PLANE LATITUDE, RADIANS', 'texmode', 'on')
      | port_label('output', 3, 'PLANE LONGITUDE, RADIANS', 'texmode', 'on')
  wires:
  Data Store Read4/1 -> SimConnect Sink1/4
  Constant4/1 -> SimConnect Sink1/2
  Constant3/1 -> SimConnect Sink1/1
  Constant1/1 -> SimConnect Sink1/7
  Constant5/1 -> SimConnect Sink1/3
  Constant/1 -> SimConnect Sink1/6
  Data Store Read5/1 -> SimConnect Sink1/5
  Constant2/1 -> SimConnect Sink1/8
  SimConnect Source1/1 -> Display3/1, Data Store Write2/1
  SimConnect Source1/2 -> Display2/1, Data Store Write/1
  SimConnect Source1/3 -> Display1/1, Data Store Write1/1
  Data Store Read1/1 -> Display11/1
  Data Store Read/1 -> Display10/1

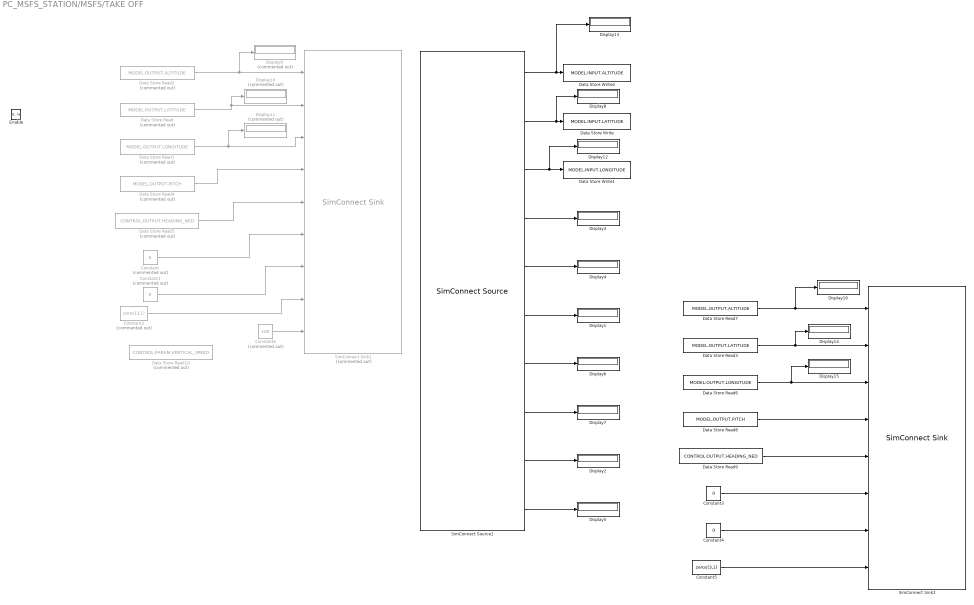
== system PC_MSFS_STATION/MSFS/TAKE OFF ==
  Enable : EnablePort
  Constant : Constant  Commented=on  Value=0  SampleTime=-1
  Constant1 : Constant  Commented=on  Value=0  SampleTime=-1
  Constant2 : Constant  Commented=on  Value=zeros(3,1)  SampleTime=-1
  Constant3 : Constant  Value=0  SampleTime=-1
  Constant4 : Constant  Value=0  SampleTime=-1
  Constant5 : Constant  Value=zeros(3,1)  SampleTime=-1
  Constant6 : Constant  Commented=on  Value=100  SampleTime=-1
  Data Store Read : DataStoreRead  Commented=on  DataStoreName=MODEL  DataStoreElements=MODEL.OUTPUT.LATITUDE  IndexOptions=Index vector (dialog)  Indices=1  OutputSizes=1
  Data Store Read1 : DataStoreRead  Commented=on  DataStoreName=MODEL  DataStoreElements=MODEL.OUTPUT.LONGITUDE  IndexOptions=Index vector (dialog)  Indices=1  OutputSizes=1
  Data Store Read10 : DataStoreRead  Commented=on  DataStoreName=CONTROL  DataStoreElements=CONTROL.PARAM.VERTICAL_SPEED  IndexOptions=Index vector (dialog)  Indices=1  OutputSizes=1
  Data Store Read2 : DataStoreRead  Commented=on  DataStoreName=MODEL  DataStoreElements=MODEL.OUTPUT.ALTITUDE  IndexOptions=Index vector (dialog)  Indices=1  OutputSizes=1
  Data Store Read3 : DataStoreRead  DataStoreName=MODEL  DataStoreElements=MODEL.OUTPUT.LATITUDE  IndexOptions=Index vector (dialog)  Indices=1  OutputSizes=1
  Data Store Read4 : DataStoreRead  Commented=on  DataStoreName=MODEL  DataStoreElements=MODEL.OUTPUT.PITCH  IndexOptions=Index vector (dialog)  Indices=1  OutputSizes=1
  Data Store Read5 : DataStoreRead  Commented=on  DataStoreName=CONTROL  DataStoreElements=CONTROL.OUTPUT.HEADING_NED  IndexOptions=Index vector (dialog)  Indices=1  OutputSizes=1
  Data Store Read6 : DataStoreRead  DataStoreName=MODEL  DataStoreElements=MODEL.OUTPUT.LONGITUDE  IndexOptions=Index vector (dialog)  Indices=1  OutputSizes=1
  Data Store Read7 : DataStoreRead  DataStoreName=MODEL  DataStoreElements=MODEL.OUTPUT.ALTITUDE  IndexOptions=Index vector (dialog)  Indices=1  OutputSizes=1
  Data Store Read8 : DataStoreRead  DataStoreName=MODEL  DataStoreElements=MODEL.OUTPUT.PITCH  IndexOptions=Index vector (dialog)  Indices=1  OutputSizes=1
  Data Store Read9 : DataStoreRead  DataStoreName=CONTROL  DataStoreElements=CONTROL.OUTPUT.HEADING_NED  IndexOptions=Index vector (dialog)  Indices=1  OutputSizes=1
  Data Store Write : DataStoreWrite  DataStoreName=MODEL  DataStoreElements=MODEL.INPUT.LATITUDE  IndexOptions=Index vector (dialog)  Indices=1  OutputSizes=1
  Data Store Write1 : DataStoreWrite  DataStoreName=MODEL  DataStoreElements=MODEL.INPUT.LONGITUDE  IndexOptions=Index vector (dialog)  Indices=1  OutputSizes=1
  Data Store Write4 : DataStoreWrite  DataStoreName=MODEL  DataStoreElements=MODEL.INPUT.ALTITUDE  IndexOptions=Index vector (dialog)  Indices=1  OutputSizes=1
  Display{1..8,12..16} (13 alike) : Display
  Display10 : Display  Commented=on
  Display11 : Display  Commented=on
  Display9 : Display  Commented=on
  SimConnect Sink1 : SimConnectToolbox/SimConnect Sink  Commented=on  configurationIndex=0  connectionName=SimConnectSink  variables=|
      | PLANE ALTITUDE, FEET;
      | PLANE LATITUDE, RADIANS;
      | PLANE LONGITUDE, RADIANS;
      | PLANE PITCH DEGREES, RADIANS;
      | PLANE HEADING DEGREES MAGNETIC, RADIANS;
      | ROTATION VELOCITY BODY X, FEET PER SECOND;
      | AILERON POSITION, POSITION;
      | AILERON TRIM PCT, PERCENT;
      | VERTICAL SPEED, FEET PER SECOND;
      settings: SourceProductName=SimConnect Toolbox
      mask Display:
      | % This is a new mask on top of the base mask.
      | % Use "View base mask" link below to see the base mask.
      | %port_label('input', 1, 'Rudder Trim', 'texmode', 'on')
      | port_label('input', 1, 'PLANE ALTITUDE, FEET', 'texmode', 'on')
      | port_label('input', 2, 'PLANE LATITUDE, RADIANS', 'texmode', 'on')
      | port_label('input', 3, 'PLANE LONGITUDE, RADIANS', 'texmode', 'on')
      | port_label('input', 4, 'PITCH DEGREES, RADIANS', 'texmode', 'on')
      | port_label('input', 5, 'HEADING DEGREES TRUE, RADIANS', 'texmode', 'on')
      | port_label('input', 6, 'VELOCITY BODY X, FEET PER SECOND', 'texmode', 'on')
      | port_label('input', 7, 'AILERON POSITION, POSITION', 'texmode', 'on')
      | port_label('input', 8, 'AILERON TRIM PCT, PERCENT OVER 100', 'texmode', 'on')
      | port_label('input', 9, 'VERTICAL SPEED, FEET PER SECOND', 'texmode', 'on')
  SimConnect Sink2 : SimConnectToolbox/SimConnect Sink  configurationIndex=0  connectionName=SimConnectSink  variables=|
      | PLANE ALTITUDE, FEET;
      | PLANE LATITUDE, RADIANS;
      | PLANE LONGITUDE, RADIANS;
      | PLANE PITCH DEGREES, RADIANS;
      | PLANE HEADING DEGREES MAGNETIC, RADIANS;
      | ROTATION VELOCITY BODY X, FEET PER SECOND;
      | AILERON POSITION, POSITION;
      | AILERON TRIM PCT, PERCENT;
      settings: SourceProductName=SimConnect Toolbox
      mask Display:
      | % This is a new mask on top of the base mask.
      | % Use "View base mask" link below to see the base mask.
      | %port_label('input', 1, 'Rudder Trim', 'texmode', 'on')
      | port_label('input', 1, 'PLANE ALTITUDE, FEET', 'texmode', 'on')
      | port_label('input', 2, 'PLANE LATITUDE, RADIANS', 'texmode', 'on')
      | port_label('input', 3, 'PLANE LONGITUDE, RADIANS', 'texmode', 'on')
      | port_label('input', 4, 'PITCH DEGREES, RADIANS', 'texmode', 'on')
      | port_label('input', 5, 'HEADING DEGREES TRUE, RADIANS', 'texmode', 'on')
      | port_label('input', 6, 'VELOCITY BODY X, FEET PER SECOND', 'texmode', 'on')
      | port_label('input', 7, 'AILERON POSITION, POSITION', 'texmode', 'on')
      | port_label('input', 8, 'AILERON TRIM PCT, PERCENT OVER 100', 'texmode', 'on')
  SimConnect Source1 : SimConnectToolbox/SimConnect Source  configurationIndex=0  connectionName=SimConnectSource  variables=|
      | PLANE ALTITUDE, FEET;
      | PLANE LATITUDE, RADIANS;
      | PLANE LONGITUDE, RADIANS;
      | ROTATION VELOCITY BODY X, FEET PER SECOND;
      | PLANE PITCH DEGREES, RADIANS;
      | PLANE HEADING DEGREES TRUE, RADIANS;
      | PLANE HEADING DEGREES MAGNETIC, RADIANS;
      | PLANE HEADING DEGREES GYRO, DEGREES;
      | AILERON POSITION, POSITION;
      | AILERON TRIM PCT, PERCENT OVER 100;
      settings: SourceProductName=SimConnect Toolbox
      mask Display:
      | % This is a new mask on top of the base mask.
      | % Use "View base mask" link below to see the base mask.
      | % port_label('output', 1, 'g', 'texmode', 'on')
      | port_label('output', 1, 'PLANE ALTITUDE, FEET', 'texmode', 'on')
      | port_label('output', 2, 'PLANE LATITUDE, RADIANS', 'texmode', 'on')
      | port_label('output', 3, 'PLANE LONGITUDE, RADIANS', 'texmode', 'on')
      | port_label('output', 4, 'VELOCITY BODY X, FEET PER SECOND', 'texmode', 'on')
      | port_label('output', 5, 'PITCH DEGREES, RADIANS', 'texmode', 'on')
      | port_label('output', 6, 'HEADING DEGREES TRUE, RADIANS', 'texmode', 'on')
      | port_label('output', 7, 'HEADING DEGREES MAGNETIC, RADIANS', 'texmode', 'on')
      | port_label('output', 8, 'HEADING DEGREES GYRO, DEGREES', 'texmode', 'on')
      | port_label('output', 9, 'AILERON POSITION, POSITION', 'texmode', 'on')
      | port_label('output', 10, 'AILERON TRIM PCT, PERCENT OVER 100', 'texmode', 'on')
  wires:
  Constant2/1 -> SimConnect Sink1/8
  SimConnect Source1/9 -> Display2/1
  Data Store Read5/1 -> SimConnect Sink1/5
  Constant/1 -> SimConnect Sink1/6
  Constant1/1 -> SimConnect Sink1/7
  SimConnect Source1/5 -> Display4/1
  SimConnect Source1/3 -> Display12/1, Data Store Write1/1
  SimConnect Source1/2 -> Display8/1, Data Store Write/1
  SimConnect Source1/8 -> Display7/1
  SimConnect Source1/6 -> Display1/1
  Data Store Read4/1 -> SimConnect Sink1/4
  SimConnect Source1/4 -> Display3/1
  SimConnect Source1/7 -> Display6/1
  SimConnect Source1/10 -> Display5/1
  Data Store Read2/1 -> SimConnect Sink1/1, Display9/1
  Data Store Read/1 -> Display10/1, SimConnect Sink1/2
  Data Store Read1/1 -> Display11/1, SimConnect Sink1/3
  SimConnect Source1/1 -> Display13/1, Data Store Write4/1
  Constant4/1 -> SimConnect Sink2/7
  Data Store Read9/1 -> SimConnect Sink2/5
  Data Store Read7/1 -> Display16/1, SimConnect Sink2/1
  Constant5/1 -> SimConnect Sink2/8
  Data Store Read8/1 -> SimConnect Sink2/4
  Data Store Read6/1 -> Display15/1, SimConnect Sink2/3
  Constant3/1 -> SimConnect Sink2/6
  Data Store Read3/1 -> Display14/1, SimConnect Sink2/2
  Constant6/1 -> SimConnect Sink1/9

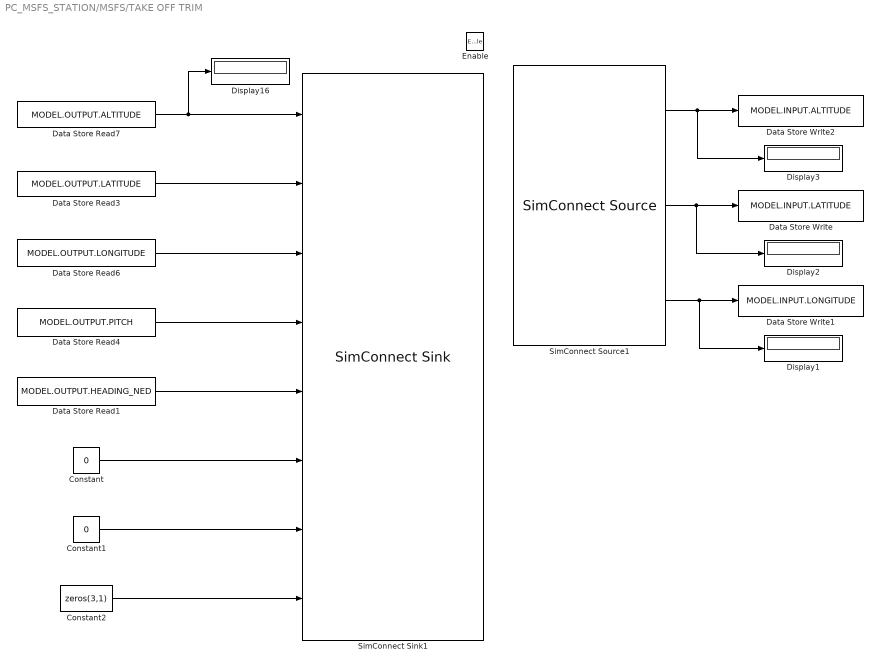
== system PC_MSFS_STATION/MSFS/TAKE OFF TRIM ==
  Enable : EnablePort
  Constant : Constant  Value=0  SampleTime=-1
  Constant1 : Constant  Value=0  SampleTime=-1
  Constant2 : Constant  Value=zeros(3,1)  SampleTime=-1
  Data Store Read1 : DataStoreRead  DataStoreName=MODEL  DataStoreElements=MODEL.OUTPUT.HEADING_NED  IndexOptions=Index vector (dialog)  Indices=1  OutputSizes=1
  Data Store Read3 : DataStoreRead  DataStoreName=MODEL  DataStoreElements=MODEL.OUTPUT.LATITUDE  IndexOptions=Index vector (dialog)  Indices=1  OutputSizes=1
  Data Store Read4 : DataStoreRead  DataStoreName=MODEL  DataStoreElements=MODEL.OUTPUT.PITCH  IndexOptions=Index vector (dialog)  Indices=1  OutputSizes=1
  Data Store Read6 : DataStoreRead  DataStoreName=MODEL  DataStoreElements=MODEL.OUTPUT.LONGITUDE  IndexOptions=Index vector (dialog)  Indices=1  OutputSizes=1
  Data Store Read7 : DataStoreRead  DataStoreName=MODEL  DataStoreElements=MODEL.OUTPUT.ALTITUDE  IndexOptions=Index vector (dialog)  Indices=1  OutputSizes=1
  Data Store Write : DataStoreWrite  DataStoreName=MODEL  DataStoreElements=MODEL.INPUT.LATITUDE  IndexOptions=Index vector (dialog)  Indices=1  OutputSizes=1
  Data Store Write1 : DataStoreWrite  DataStoreName=MODEL  DataStoreElements=MODEL.INPUT.LONGITUDE  IndexOptions=Index vector (dialog)  Indices=1  OutputSizes=1
  Data Store Write2 : DataStoreWrite  DataStoreName=MODEL  DataStoreElements=MODEL.INPUT.ALTITUDE  IndexOptions=Index vector (dialog)  Indices=1  OutputSizes=1
  Display{1..3,16} (4 alike) : Display
  SimConnect Sink1 : SimConnectToolbox/SimConnect Sink  configurationIndex=0  connectionName=SimConnectSink  variables=|
      | PLANE ALTITUDE, FEET;
      | PLANE LATITUDE, RADIANS;
      | PLANE LONGITUDE, RADIANS;
      | PLANE PITCH DEGREES, RADIANS;
      | PLANE HEADING DEGREES TRUE, RADIANS;
      | ROTATION VELOCITY BODY X, FEET PER SECOND;
      | AILERON POSITION, POSITION;
      | AILERON TRIM PCT, PERCENT;
      settings: SourceProductName=SimConnect Toolbox
      mask Display:
      | % This is a new mask on top of the base mask.
      | % Use "View base mask" link below to see the base mask.
      | %port_label('input', 1, 'Rudder Trim', 'texmode', 'on')
      | port_label('input', 1, 'PLANE ALTITUDE, FEET', 'texmode', 'on')
      | port_label('input', 2, 'PLANE LATITUDE, RADIANS', 'texmode', 'on')
      | port_label('input', 3, 'PLANE LONGITUDE, RADIANS', 'texmode', 'on')
      | port_label('input', 4, 'PITCH DEGREES, RADIANS', 'texmode', 'on')
      | port_label('input', 5, 'HEADING DEGREES TRUE, RADIANS', 'texmode', 'on')
      | port_label('input', 6, 'VELOCITY BODY X, FEET PER SECOND', 'texmode', 'on')
      | port_label('input', 7, 'AILERON POSITION, POSITION', 'texmode', 'on')
      | port_label('input', 8, 'AILERON TRIM PCT, PERCENT OVER 100', 'texmode', 'on')
  SimConnect Source1 : SimConnectToolbox/SimConnect Source  configurationIndex=0  connectionName=SimConnectSource  variables=|
      | PLANE ALTITUDE, FEET;
      | PLANE LATITUDE, RADIANS;
      | PLANE LONGITUDE, RADIANS;
      settings: SourceProductName=SimConnect Toolbox
      mask Display:
      | % This is a new mask on top of the base mask.
      | % Use "View base mask" link below to see the base mask.
      | % port_label('output', 1, 'g', 'texmode', 'on')
      | port_label('output', 1, 'PLANE ALTITUDE, FEET', 'texmode', 'on')
      | port_label('output', 2, 'PLANE LATITUDE, RADIANS', 'texmode', 'on')
      | port_label('output', 3, 'PLANE LONGITUDE, RADIANS', 'texmode', 'on')
  wires:
  Data Store Read7/1 -> SimConnect Sink1/1, Display16/1
  SimConnect Source1/2 -> Data Store Write/1, Display2/1
  SimConnect Source1/1 -> Display3/1, Data Store Write2/1
  SimConnect Source1/3 -> Display1/1, Data Store Write1/1
  Data Store Read3/1 -> SimConnect Sink1/2
  Data Store Read6/1 -> SimConnect Sink1/3
  Data Store Read1/1 -> SimConnect Sink1/5
  Constant1/1 -> SimConnect Sink1/7
  Constant/1 -> SimConnect Sink1/6
  Constant2/1 -> SimConnect Sink1/8
  Data Store Read4/1 -> SimConnect Sink1/4

== matlab function PC_MSFS_STATION/CONTROL/CONTROL UPDATE ==
  data: CONTROL_IN input; CONTROL output Bus: CONTROL_Bus; STATE input; ALTITUDE input
function CONTROL = CONTROL_UPDATE(CONTROL_IN, STATE, ALTITUDE)
% COPY CONTROL BUS
CONTROL = CONTROL_IN;
CONTROL.PARAM.SIM_TIME = CONTROL.PARAM.SIM_TIME + CONTROL.PARAM.SAMPLING_TIME;
curr_sim_time = CONTROL.PARAM.SIM_TIME;
deltat = CONTROL.PARAM.SAMPLING_TIME;
flight_status = CONTROL.PARAM.FLIGHT_STATUS;
timer = CONTROL.PARAM.TIMER;

at_wp = CONTROL.OUTPUT.AT_WP;
wp_flag = CONTROL.OUTPUT.ALMOST_WP;
prev_wp1 = CONTROL.PARAM.PREV_WP1;
prev_wp2 = CONTROL.PARAM.PREV_WP2;
%--------------------------------------------------------------------------
% CONTROL PARAMETERS
%--------------------------------------------------------------------------
% Nominal Control Parameters
kyd = CONTROL.PARAM.NAV_D_1;

% Navigation Variables
altitude = ALTITUDE;
altitude_control = CONTROL.PARAM.ALTITUDE;
rho = altitude + 20.902e6;

% Extra Parameters
tau_max = CONTROL.PARAM.TAU_MAX;
dist_Goal = CONTROL.PARAM.DIST_GOAL;
%--------------------------------------------------------------------------
% CONTROL TARGETS
%--------------------------------------------------------------------------
wp_index = CONTROL.TARGET.WP_INDEX;
simu_end = CONTROL.TARGET.SIMU_END;
target_latitude = CONTROL.TARGET.LATITUDE*pi/180;
target_longitude = CONTROL.TARGET.LONGITUDE*pi/180;
snom = CONTROL.TARGET.VELOCITY;
%--------------------------------------------------------------------------
% SYSTEM CURRENT STATE
%--------------------------------------------------------------------------
% Update Current State
y1 = STATE(1);
y2 = STATE(2);
vy1 = STATE(3);
vy2 = STATE(4);

% FLIGHT STATUS 0 = INITIALIZATION
if flight_status == 0
    % VIRTUAL NOMINAL CONTROLLER (tau1, tau2)
    tau1_nom_PD = - kyd*(vy1 - 0);
    tau2_nom_PD = - kyd*(vy2 - 0);
    tau1_applied = tau1_nom_PD;
    tau2_applied = tau2_nom_PD;
    
    if abs(tau1_applied) >= tau_max
        tau1_applied = sign(tau1_applied)*tau_max;
    else
        tau1_applied = tau1_applied;
    end
    
    if abs(tau2_applied) >= tau_max
        tau2_applied = sign(tau2_applied)*tau_max;
    else
        tau2_applied = tau2_applied;
    end
    if curr_sim_time >= 3
        flight_status = 2;
        timer = 0;
    end 

elseif flight_status == 1
    altitude = altitude_control;
    rho = altitude + 20.902e6;
    tau1_nom_PD = - kyd*(vy1 - 0);
    tau2_nom_PD = - kyd*(vy2 - 0);
    tau1_applied = tau1_nom_PD;
    tau2_applied = tau2_nom_PD;
    
    if abs(tau1_applied) >= tau_max
        tau1_applied = sign(tau1_applied)*tau_max;
    else
        tau1_applied = tau1_applied;
    end
    
    if abs(tau2_applied) >= tau_max
        tau2_applied = sign(tau2_applied)*tau_max;
    else
        tau2_applied = tau2_applied;
    end
    if curr_sim_time >= 10
        flight_status = 2;
        timer = 0;
    end
else
    % ON FLIGHT
    %--------------------------------------------------------------------------
    % DERIVATIVE (D) CONTROL
    %--------------------------------------------------------------------------
    altitude = altitude_control;
    rho = altitude + 20.902e6; 
    timer = timer + deltat;

    wp1 = rho*cos(target_latitude)*cos(target_longitude);
    wp2 = rho*cos(target_latitude)*sin(target_longitude);
    
    if (timer < 2*deltat)
        prev_wp1 = wp1;
        prev_wp2 = wp2;
        CONTROL.PARAM.PREV_WP1 = wp1;
        CONTROL.PARAM.PREV_WP2 = wp2;
    end

    % NOMINAL CONTROLLER
    % System Quadrant
    pos1_PD = wp1 - y1;
    pos2_PD = wp2 - y2;

    if pos1_PD >=0
        % First or fourth quadrant
        if pos2_PD >=0
            %First quadrant
            theta_PD = atan(abs(pos2_PD)/abs(pos1_PD));
        else
            % Fourth quadrant
            %                 theta_PD = 2*pi - atan(abs(pos2_PD)/abs(pos1_PD));
            theta_PD = - atan(abs(pos2_PD)/abs(pos1_PD));
        end
    else
        % Second or third quadrant
        if pos2_PD >=0
            % Second quadrant
            theta_PD = pi - atan(abs(pos2_PD)/abs(pos1_PD));
        else
            % Third quadrant
            theta_PD = pi + atan(abs(pos2_PD)/abs(pos1_PD));
        end
    end

    % New target velocity
    vs1_PD = snom*cos(theta_PD);
    vs2_PD = snom*sin(theta_PD);

    % VIRTUAL NOMINAL CONTROLLER (tau1, tau2)
    tau1_nom_PD = - kyd*(vy1 - vs1_PD);
    tau2_nom_PD = - kyd*(vy2 - vs2_PD);
    tau1_applied = tau1_nom_PD;
    tau2_applied = tau2_nom_PD;

    if abs(tau1_applied) >= tau_max
        tau1_applied = sign(tau1_applied)*tau_max;
    else
        tau1_applied = tau1_applied;
    end

    if abs(tau2_applied) >= tau_max
        tau2_applied = sign(tau2_applied)*tau_max;
    else
        tau2_applied = tau2_applied;
    end
    
    % UPDATE WP FLAG
    if (((y1 - wp1)^2 < (10*100*dist_Goal)^2)&&((y2 - wp2)^2 < (10*100*dist_Goal)^2))
%     if ((y1 - wp1)^2 + (y2 - wp2)^2 < (1000*dist_Goal)^2)
        wp_flag = 1;
    end
    
    % UPDATE TARGET WAYPOINT
    if (((y1 - wp1)^2 < dist_Goal^2)&&((y2 - wp2)^2 < dist_Goal^2))
        at_wp = 1;
        CONTROL.PARAM.PREV_WP1 = wp1;
        CONTROL.PARAM.PREV_WP2 = wp2;
    end

    if ((prev_wp1 ~= wp1)||(prev_wp2 ~= wp2))
        at_wp = 0;
        wp_flag = 0;
    end



end


%%%%%%%%%%%%%%%%%%%%%%%%%%%%%%%%%%%%%%%%%%%%%%%%%%%%%%%%%%%%%%%%%%%%%%%%%%%
% OUTPUT BUS
%%%%%%%%%%%%%%%%%%%%%%%%%%%%%%%%%%%%%%%%%%%%%%%%%%%%%%%%%%%%%%%%%%%%%%%%%%%
CONTROL.TARGET.WP_INDEX = wp_index;
CONTROL.TARGET.SIMU_END = simu_end;
CONTROL.OUTPUT.TAU1 = tau1_applied;
CONTROL.OUTPUT.TAU2 = tau2_applied;

CONTROL.PARAM.FLIGHT_STATUS = flight_status;
CONTROL.PARAM.ALTITUDE = altitude;
CONTROL.PARAM.RHO = rho;
CONTROL.PARAM.TIMER = timer;

CONTROL.OUTPUT.AT_WP = at_wp;
CONTROL.OUTPUT.ALMOST_WP = wp_flag;
return
